simulink model "ofdm_tx"  (R2023b)
settings: Solver=FixedStepAuto  StartTime=0.0  StopTime=inf  FixedStep=frameLen/Fs  RelTol=1e-3
values from neighbouring files (symbols this model uses):
  frameLen = preambleLen + ofdmLen    (= 1008)    [parameter.m]
  Fs = 1e6    (= 1000000)    [offline_analyze_rx_raw.m]    (also in parameter.m)
  payloadIdx = randi([0 M-1], numDataSC*(numOFDMSym-1), 1)    [offline_analyze_rx_demod.m]    (also in parameter.m = randi([0 M-1], numDataSC*numPayloadSym, 1); sim_ofdm_complex.m = randi([0 cfg.M-1], numDataSC*cfg.numPayloadSym, 1))
  pilotSym = ones(4, numOFDMSym)    [parameter.m]    (also in sim_ofdm_complex.m = ones(numel(cfg.pilotIdx), cfg.numOFDMSym))
  preamble = [preHalf; preHalf]    [offline_analyze_rx_raw.m]    (also in parameter.m; sim_ofdm_complex.m; sync_cfo.m)
  trainSym = pskmod(trainIdx, M, pi/4, 'gray')    [equalize_payload.m]    (also in offline_analyze_rx_demod.m = pskmod(trainIdx, M, phaseOffset, 'gray'); parameter.m; sim_ofdm_complex.m = pskmod(trainIdx, cfg.M, cfg.phaseOffset, 'gray'))
  txScale = 0.15    [parameter.m]
undefined symbols (not defined in the file or in its folder): ip
libraries: plutoradiolib x1, commofdm x1, commdigbbndpm3 x1
settings Model: Creator=yuezh  LastModifiedBy=yuezh

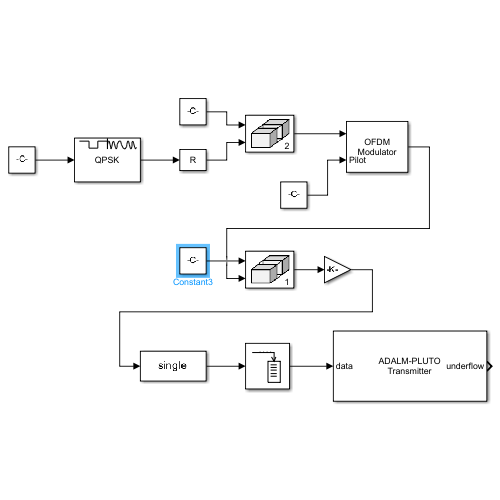
[thumbnail: Simulink's stored preview of the top-level diagram]
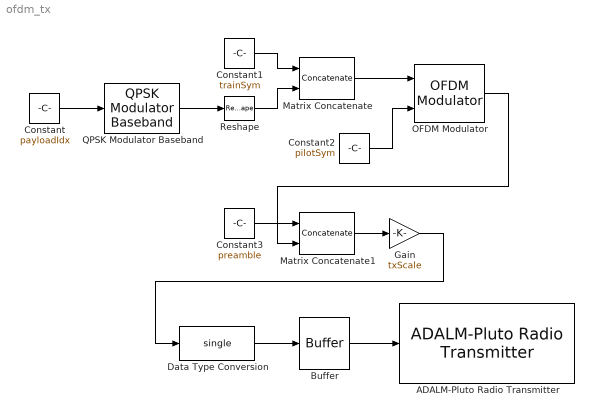
== system ofdm_tx ==
  ADALM-Pluto Radio Transmitter : plutoradiolib/ADALM-Pluto Radio Transmitter  RadioID=ip:192.168.1.10  uri=ip:10.0.0.200  CenterFrequencySource=Dialog  CenterFrequency=Fc  GainSource=Dialog  Gain=-30  ChannelMapping=1  BasebandSampleRate=Fs  UnderflowOutputPort=on  ShowAdvancedProperties=off  UseCustomFilter=off  filtPathRates=[737280000 11520000 3840000 1920000 960000 240000]  filtCoefficients=[-192 82 85 -215 228 -102 -110 290 -318 145 160 -426 471 -215 -238 633 -697 318 349 -923 1009 -457 -498 1309 -1423 640 693 -1812 1959 -876 -945 2458 -2647 1180 1268 -3290 3534 -1572 -1688 4375 -4698 2091 2247 -5836 6284 -2807 -3031 7918 -8588 3870 4225 -11182 12324 -5662 -6330 17255 -19735 9507 11312 -33568 43355 -25227 -42139 305542 305542 -42139 -25227 43355 -33568 11312 9507 -19735 17255 -6330 -5662 12324 -11182 4225 3870 -8588 7918 -3031 -2807 6284 -5836 2247 2091 -4698 4375 -1688 -1572 3534 -3290 1268 1180 -2647 2458 -945 -876 1959 -1812 693 640 -1423 1309 -498 -457 1009 -923 349 318 -697 633 -238 -215 471 -426 160 145 -318 290 -110 -102 228 -215 85 82 -192]  filtCoefficientSize=128  filtDecimInterpFactor=4  filtGain=-12  filtRFBandwidth=18000000  filterConfigStruct=struct()  DataSourceSelect=Input Port  DDSTone1Freq=5e3  DDSTone2Freq=10e3  DDSTone1Scale=0.5  DDSTone2Scale=0.25  DataTimeout=Inf  FrequencyCorrection=0  ENSMPinControlMode=None  BISTLoopbackMode=Disabled  BISTToneInject=Disabled  BISTSignalGen=PRBS  BISTToneFreq=Fs/32  BISTToneLevel=0
  Buffer : Buffer  N=10080  OutputFrames=off
  Constant : Constant  Value=payloadIdx  SampleTime=frameLen/Fs
  Constant1 : Constant  Value=trainSym  SampleTime=frameLen/Fs
  Constant2 : Constant  Value=pilotSym  SampleTime=frameLen/Fs
  Constant3 : Constant  Value=preamble  SampleTime=frameLen/Fs
  Data Type Conversion : DataTypeConversion  OutDataTypeStr=single  SaturateOnIntegerOverflow=off  RndMeth=Floor
  Gain : Gain  Gain=txScale
  Matrix Concatenate : Concatenate  Mode=Multidimensional array  ConcatenateDimension=2
  Matrix Concatenate1 : Concatenate  Mode=Multidimensional array
  OFDM Modulator : commofdm/OFDM Modulator  StatePerturbationForJacobian=1.0e-05  FFTLength=64  NumGuardBandCarriers=[6; 5]  InsertDCNull=on  PilotInputPort=on  PilotCarrierIndices=[12; 26; 40; 54]  CyclicPrefixLength=16  Windowing=off  WindowLength=1  OversamplingFactor=1  NumSymbols=11  NumTransmitAntennas=1  SimulateUsing=Interpreted execution
  QPSK Modulator Baseband : commdigbbndpm3/QPSK Modulator Baseband  InType=Integer  Enc=Gray  Ph=pi/4  outDtype=double  outWordLen=16  outUDDataType=sfix(16)  outFracLenMode=Best precision  outFracLen=15  outDataTypeStr=double  outLastDataTypeStr=double
  Reshape : Reshape  OutputDimensionality=Customize  OutputDimensions=[48,10]
  wires:
  Constant/1 -> QPSK Modulator Baseband/1
  QPSK Modulator Baseband/1 -> Reshape/1
  Matrix Concatenate/1 -> OFDM Modulator/1
  Constant2/1 -> OFDM Modulator/2
  Matrix Concatenate1/1 -> Gain/1
  Gain/1 -> Data Type Conversion/1
  Constant1/1 -> Matrix Concatenate/1
  Reshape/1 -> Matrix Concatenate/2
  Constant3/1 -> Matrix Concatenate1/1
  OFDM Modulator/1 -> Matrix Concatenate1/2
  Data Type Conversion/1 -> Buffer/1
  Buffer/1 -> ADALM-Pluto Radio Transmitter/1
